simulink model "Lab1_ContiniousMdl_and_DiscrCtrl_"  (R2013b)
settings: Solver=ode3  SolverMode=SingleTasking  StartTime=0.0  StopTime=100.0  FixedStep=10e-3  RelTol=1e-3
values from neighbouring files (symbols this model uses):
  Adk = Ad - Bd*K    [Lab1.m]
  K = place(Ad,Bd,Rp)    [Lab1.m]
undefined symbols (not defined in the file or in its folder): A, B, Bd, C, Cd, Dd
settings Model: Creator=user  LastModifiedBy=user
settings DataIOCC: LimitDataPoints=off

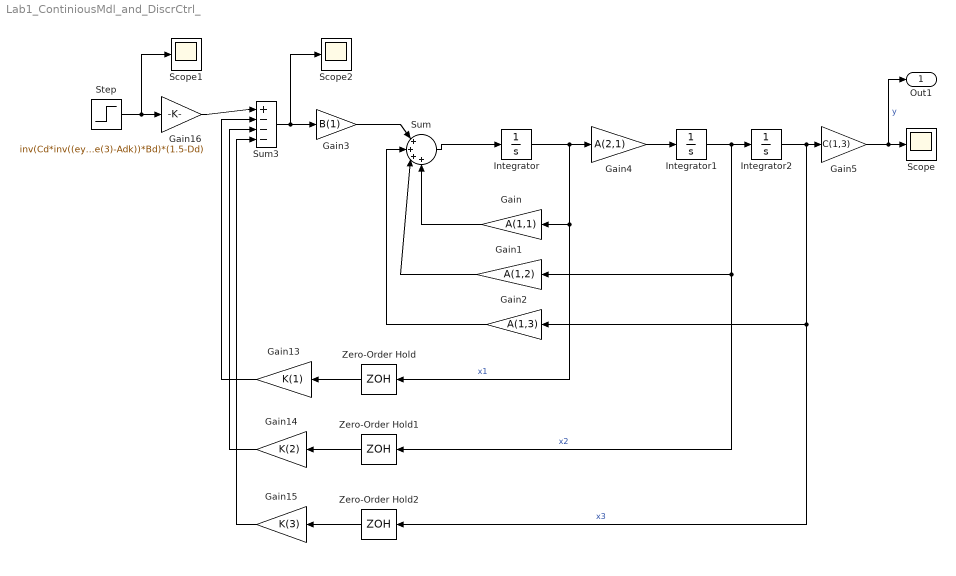
== system Lab1_ContiniousMdl_and_DiscrCtrl_ ==
  Gain : Gain  Gain=A(1,1)
  Gain1 : Gain  Gain=A(1,2)
  Gain13 : Gain  Gain=K(1)
  Gain14 : Gain  Gain=K(2)
  Gain15 : Gain  Gain=K(3)
  Gain16 : Gain  Gain=inv(Cd*inv((eye(3)-Adk))*Bd)*(1.5-Dd)
  Gain2 : Gain  Gain=A(1,3)
  Gain3 : Gain  Gain=B(1)
  Gain4 : Gain  Gain=A(2,1)
  Gain5 : Gain  Gain=C(1,3)
  Integrator : Integrator
  Integrator1 : Integrator
  Integrator2 : Integrator
  Scope : Scope
      settings: SaveName=ContMdl_out
  Scope1 : Scope
      settings: SaveName=SetPoint
  Scope2 : Scope
      settings: SaveName=SetPoint1
  Step : Step  Time=0  SampleTime=0.4
  Sum : Sum  Inputs=|++++
  Sum3 : Sum  Inputs=|+---
  Zero-Order Hold : ZeroOrderHold  SampleTime=0.4
  Zero-Order Hold1 : ZeroOrderHold  SampleTime=0.4
  Zero-Order Hold2 : ZeroOrderHold  SampleTime=0.4
  Out1 : Outport
  wires:
  Sum/1 -> Integrator/1
  Gain/1 -> Sum/4
  Gain4/1 -> Integrator1/1
  Gain1/1 -> Sum/3
  Gain2/1 -> Sum/2
  Gain3/1 -> Sum/1
  Gain5/1 -> Out1/1, Scope/1  "y"
  Integrator/1 -> Gain4/1, Zero-Order Hold/1, Gain/1  "x1"
  Integrator1/1 -> Zero-Order Hold1/1, Gain1/1, Integrator2/1  "x2"
  Integrator2/1 -> Zero-Order Hold2/1, Gain2/1, Gain5/1  "x3"
  Step/1 -> Scope1/1, Gain16/1
  Gain13/1 -> Sum3/2
  Gain14/1 -> Sum3/3
  Gain15/1 -> Sum3/4
  Zero-Order Hold/1 -> Gain13/1
  Zero-Order Hold1/1 -> Gain14/1
  Zero-Order Hold2/1 -> Gain15/1
  Gain16/1 -> Sum3/1
  Sum3/1 -> Scope2/1, Gain3/1
